simulink model "REG0_NELINEARIZOVANE_simulink"  (R2019b)
settings: Solver=FixedStepAuto  StartTime=0.0  StopTime=5  FixedStep=0.01  MaxStep=0.01  RelTol=1e-3
values from neighbouring files (symbols this model uses):
  a = 0.5    [MSM_skript.m]    (also in matlab.mat; stavovaRovnice.m)
  b = 0.75    [MSM_skript.m]    (also in matlab.mat; stavovaRovnice.m)
  b1 = 6.1    [MSM_skript.m]    (also in matlab.mat; stavovaRovnice.m)
  b2 = 8.8    [MSM_skript.m]    (also in matlab.mat; stavovaRovnice.m)
  c = 1.25    [MSM_skript.m]    (also in matlab.mat; stavovaRovnice.m)
  d = 1    [MSM_skript.m]    (also in matlab.mat; stavovaRovnice.m)
  G1 = m1*g    (= 49.05)    [MSM_skript.m]    (also in matlab.mat = 9.81; stavovaRovnice.m)
  G2 = m2*g    (= 19.62)    [MSM_skript.m]    (also in matlab.mat = 9.81; stavovaRovnice.m)
  I1 = m1*b^2    (= 2.8125)    [stavovaRovnice.m]
  I2 = m2*c^2    (= 3.125)    [stavovaRovnice.m]
  k = 5.8*100    (= 580)    [MSM_skript.m]    (also in matlab.mat; stavovaRovnice.m)
  kt = 1.1*100    (= 110)    [MSM_skript.m]    (also in matlab.mat; stavovaRovnice.m)
  x10 = phi10    [MSM_skript.m]    (also in matlab.mat = 0.261799387799; stavovaRovnice.m)
  x20 = dphi10    (= 0)    [MSM_skript.m]    (also in matlab.mat; stavovaRovnice.m)
  x30 = phi20    (= 0)    [MSM_skript.m]    (also in matlab.mat; stavovaRovnice.m)
  x40 = dphi20    (= 0)    [MSM_skript.m]    (also in matlab.mat; stavovaRovnice.m)
undefined symbols (not defined in the file or in its folder): Kr0
settings Model: Creator=jakub  LastModifiedBy=jakub

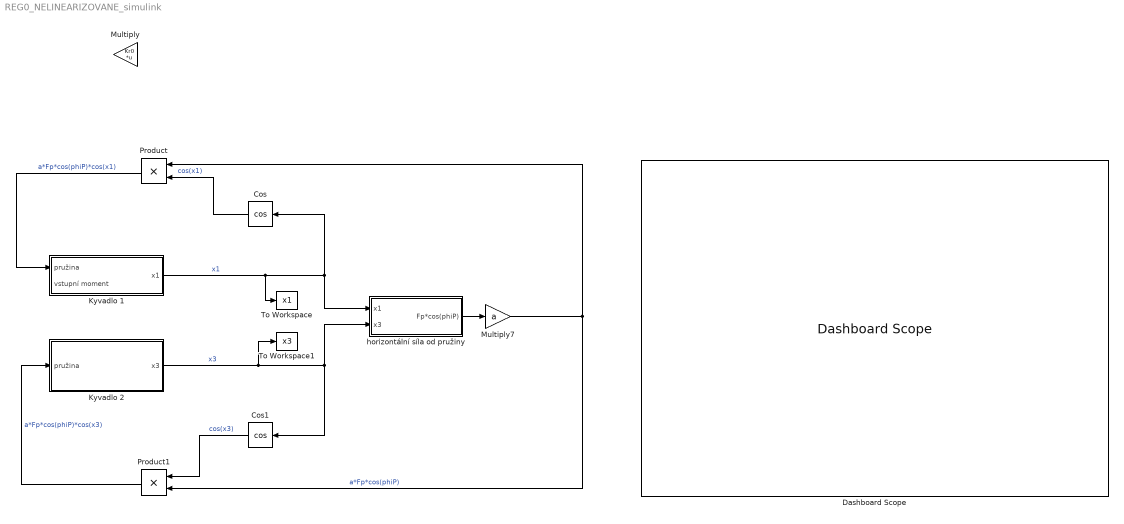
== system REG0_NELINEARIZOVANE_simulink ==
  Cos : Trigonometry  Operator=cos
  Cos1 : Trigonometry  Operator=cos
  Dashboard Scope : DashboardScope  Ymin=-1  Ymax=1
  Kyvadlo 1 : Subsystem
  Kyvadlo 2 : Subsystem
  Multiply : Gain  Gain=Kr0  Multiplication=Matrix(K*u) (u vector)
  Multiply7 : Gain  Gain=a
  Product : Product
  Product1 : Product
  To Workspace : ToWorkspace  VariableName=x1  SaveFormat=Timeseries  SampleTime=-1
      settings: Save2DSignal=2-D array (concatenate along first dimension)
  To Workspace1 : ToWorkspace  VariableName=x3  SaveFormat=Timeseries  SampleTime=-1
      settings: Save2DSignal=2-D array (concatenate along first dimension)
  horizontální síla od pružiny : Subsystem
  wires:
  Cos/1 -> Product/2  "cos(x1)"
  horizontální síla od pružiny/1(Fp*cos(phiP)) -> Multiply7/1
  Multiply7/1 -> Product1/2, Product/1  "a*Fp*cos(phiP)"
  Cos1/1 -> Product1/1  "cos(x3)"
  Kyvadlo 1/1(x1) -> To Workspace/1, horizontální síla od pružiny/1(x1), Cos/1  "x1"
  Product/1 -> Kyvadlo 1/1(pružina)  "a*Fp*cos(phiP)*cos(x1)"
  ? -> Kyvadlo 1/2(vstupní moment)
  Kyvadlo 2/1(x3) -> To Workspace1/1, horizontální síla od pružiny/2(x3), Cos1/1  "x3"
  Product1/1 -> Kyvadlo 2/1(pružina)  "a*Fp*cos(phiP)*cos(x3)"

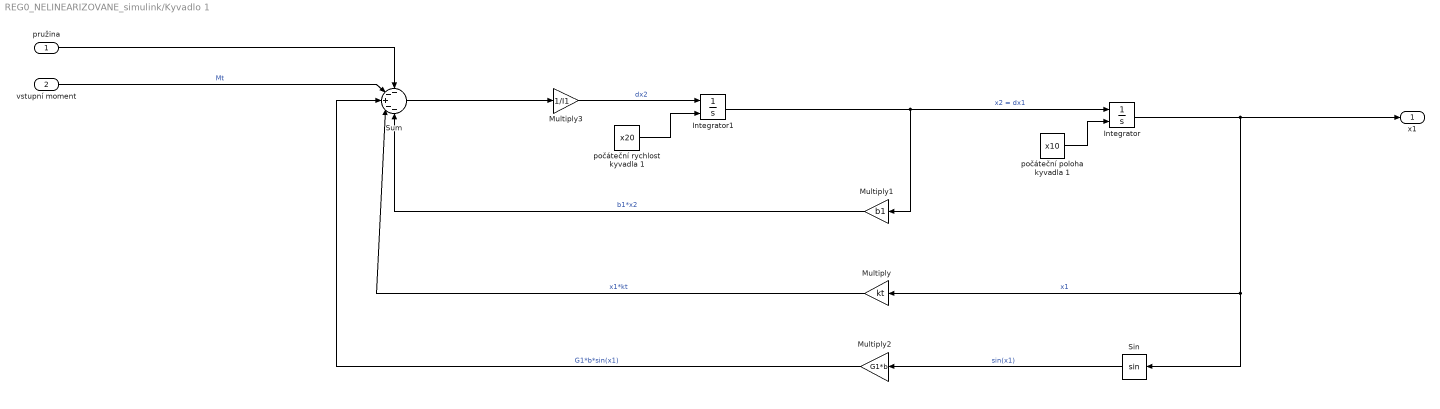
== system REG0_NELINEARIZOVANE_simulink/Kyvadlo 1 ==
  pružina : Inport
  vstupní moment : Inport  Port=2
  Integrator : Integrator  InitialConditionSource=external
  Integrator1 : Integrator  InitialConditionSource=external
  Multiply : Gain  Gain=kt
  Multiply1 : Gain  Gain=b1
  Multiply2 : Gain  Gain=G1*b
  Multiply3 : Gain  Gain=1/I1
  Sin : Trigonometry
  Sum : Sum  Inputs=--+--
  počáteční poloha kyvadla 1 : Constant  Value=x10
  počáteční rychlost kyvadla 1 : Constant  Value=x20
  x1 : Outport
  wires:
  Multiply2/1 -> Sum/3  "G1*b*sin(x1)"
  počáteční poloha kyvadla 1/1 -> Integrator/2
  Sum/1 -> Multiply3/1
  Sin/1 -> Multiply2/1  "sin(x1)"
  Multiply3/1 -> Integrator1/1  "dx2"
  vstupní moment/1 -> Sum/2  "Mt"
  Integrator1/1 -> Integrator/1, Multiply1/1  "x2 = dx1"
  Multiply/1 -> Sum/4  "x1*kt"
  Multiply1/1 -> Sum/5  "b1*x2"
  pružina/1 -> Sum/1
  počáteční rychlost kyvadla 1/1 -> Integrator1/2
  Integrator/1 -> Sin/1, Multiply/1, x1/1  "x1"

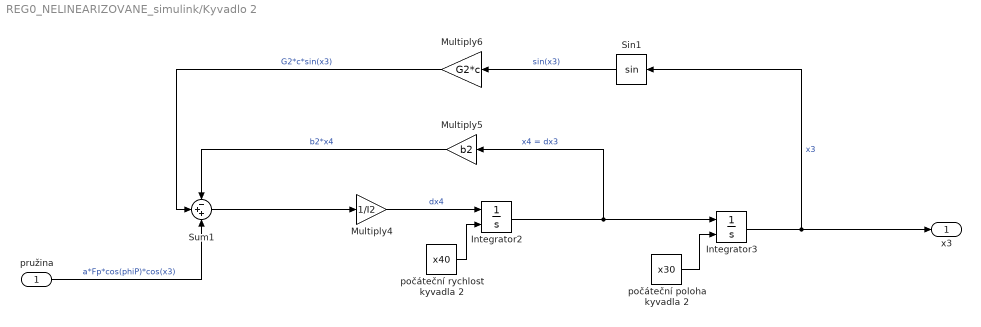
== system REG0_NELINEARIZOVANE_simulink/Kyvadlo 2 ==
  pružina : Inport
  Integrator2 : Integrator  InitialConditionSource=external
  Integrator3 : Integrator  InitialConditionSource=external
  Multiply4 : Gain  Gain=1/I2
  Multiply5 : Gain  Gain=b2
  Multiply6 : Gain  Gain=G2*c
  Sin1 : Trigonometry
  Sum1 : Sum  Inputs=-++
  počáteční poloha kyvadla 2 : Constant  Value=x30
  počáteční rychlost kyvadla 2 : Constant  Value=x40
  x3 : Outport
  wires:
  Multiply4/1 -> Integrator2/1  "dx4"
  Multiply5/1 -> Sum1/1  "b2*x4"
  Multiply6/1 -> Sum1/2  "G2*c*sin(x3)"
  Sin1/1 -> Multiply6/1  "sin(x3)"
  pružina/1 -> Sum1/3  "a*Fp*cos(phiP)*cos(x3)"
  Sum1/1 -> Multiply4/1
  počáteční poloha kyvadla 2/1 -> Integrator3/2
  Integrator3/1 -> x3/1, Sin1/1  "x3"
  počáteční rychlost kyvadla 2/1 -> Integrator2/2
  Integrator2/1 -> Integrator3/1, Multiply5/1  "x4 = dx3"

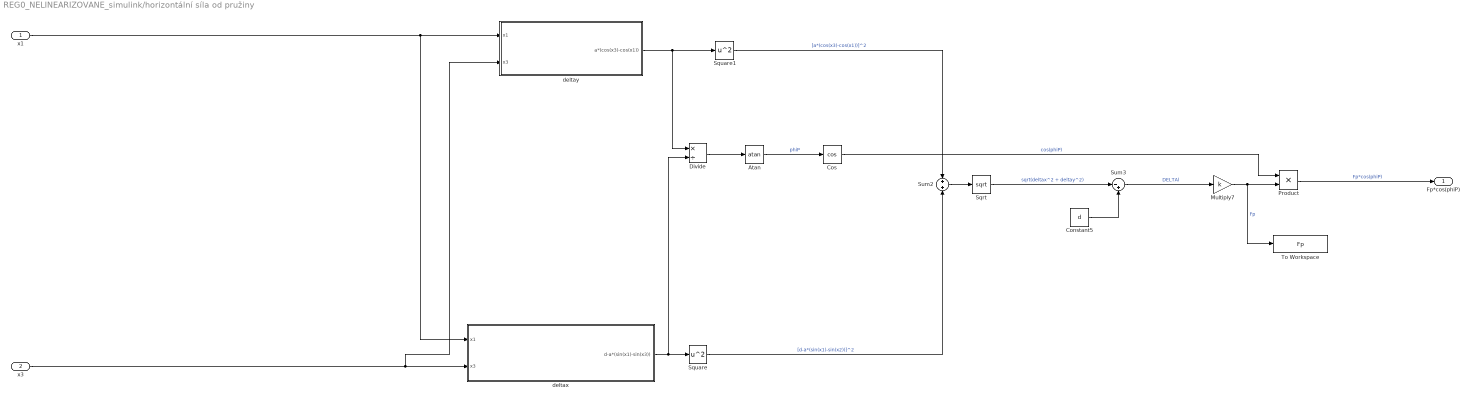
== system REG0_NELINEARIZOVANE_simulink/horizontální síla od pružiny ==
  x1 : Inport
  x3 : Inport  Port=2
  Atan : Trigonometry  Operator=atan
  Constant5 : Constant  Value=d
  Cos : Trigonometry  Operator=cos
  Divide : Product  Inputs=*/
  Multiply7 : Gain  Gain=k
  Product : Product
  Sqrt : Sqrt  SaturateOnIntegerOverflow=on
  Square : Math  Operator=square  SignedPower=off  SaturateOnIntegerOverflow=on
  Square1 : Math  Operator=square  SignedPower=off  SaturateOnIntegerOverflow=on
  Sum2 : Sum  Inputs=+|+
  Sum3 : Sum  Inputs=|-+
  To Workspace : ToWorkspace  VariableName=Fp  SaveFormat=Timeseries  SampleTime=-1
  deltax : Subsystem
  deltay : Subsystem
  Fp*cos(phiP) : Outport
  wires:
  Product/1 -> Fp*cos(phiP)/1  "Fp*cos(phiP)"
  Cos/1 -> Product/1  "cos(phiP)"
  Constant5/1 -> Sum3/2
  Multiply7/1 -> To Workspace/1, Product/2  "Fp"
  Sqrt/1 -> Sum3/1  "sqrt(deltax^2 + deltay^2)"
  Sum3/1 -> Multiply7/1  "DELTAl"
  deltay/1(a*(cos(x3)-cos(x1))) -> Divide/1, Square1/1
  deltax/1(d-a*(sin(x1)-sin(x3))) -> Divide/2, Square/1
  Sum2/1 -> Sqrt/1
  Divide/1 -> Atan/1
  x3/1 -> deltay/2(x3), deltax/2(x3)
  Square1/1 -> Sum2/1  "[a*(cos(x3)-cos(x1))]^2"
  Square/1 -> Sum2/2  "[d-a*(sin(x1)-sin(x2))]^2"
  x1/1 -> deltax/1(x1), deltay/1(x1)
  Atan/1 -> Cos/1  "phiP"

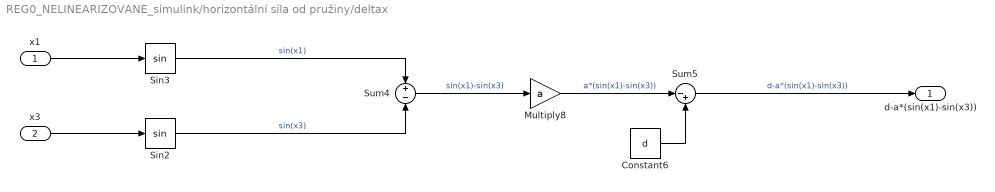
== system REG0_NELINEARIZOVANE_simulink/horizontální síla od pružiny/deltax ==
  x1 : Inport
  x3 : Inport  Port=2
  Constant6 : Constant  Value=d
  Multiply8 : Gain  Gain=a
  Sin2 : Trigonometry
  Sin3 : Trigonometry
  Sum4 : Sum  Inputs=+|-
  Sum5 : Sum  Inputs=|-+
  d-a*(sin(x1)-sin(x3)) : Outport
  wires:
  Sin2/1 -> Sum4/2  "sin(x3)"
  Sum5/1 -> d-a*(sin(x1)-sin(x3))/1  "d-a*(sin(x1)-sin(x3))"
  Sin3/1 -> Sum4/1  "sin(x1)"
  Constant6/1 -> Sum5/2
  x3/1 -> Sin2/1
  Sum4/1 -> Multiply8/1  "sin(x1)-sin(x3)"
  x1/1 -> Sin3/1
  Multiply8/1 -> Sum5/1  "a*(sin(x1)-sin(x3))"

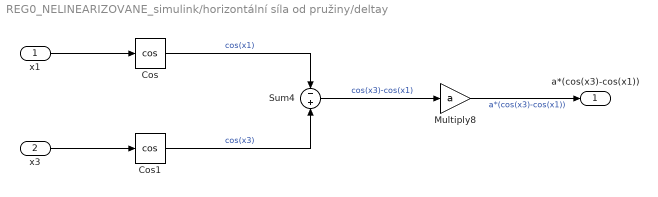
== system REG0_NELINEARIZOVANE_simulink/horizontální síla od pružiny/deltay ==
  x1 : Inport
  x3 : Inport  Port=2
  Cos : Trigonometry  Operator=cos
  Cos1 : Trigonometry  Operator=cos
  Multiply8 : Gain  Gain=a
  Sum4 : Sum  Inputs=-|+
  a*(cos(x3)-cos(x1)) : Outport
  wires:
  x3/1 -> Cos1/1
  Multiply8/1 -> a*(cos(x3)-cos(x1))/1  "a*(cos(x3)-cos(x1))"
  Cos/1 -> Sum4/1  "cos(x1)"
  x1/1 -> Cos/1
  Sum4/1 -> Multiply8/1  "cos(x3)-cos(x1)"
  Cos1/1 -> Sum4/2  "cos(x3)"
